simulink model "ArduinoUnoTemplate"  (R2021b)
settings: Solver=ode3  StartTime=0.0  StopTime=10  RelTol=1e-3  EnableMultiTasking=on
libraries: simulink x1, arduinolib x1
settings Model: FPTRunName=Active  ExtModeTrigDuration=2  Creator=cirie  LastModifiedBy=cirie
settings SolverCC: AlgebraicLoopSolver=TrustRegion
settings DataIOCC: LimitDataPoints=on  SaveFormat=Array
settings OptimizationCC: ExpressionDepthLimit=2147483647  LifeSpan=Inf  MaxStackSize=64
settings DebuggingCC: UnderspecifiedInitializationDetection=Classic  MergeDetectMultiDrivingBlocksExec=none  FcnCallInpInsideContextMsg=warning  AllowSymbolicDim=off  StateNameClashWarn=warning  SFUnexpectedBacktrackingDiag=warning  SFNoUnconditionalDefaultTransitionDiag=warning  SFExecutionAtInitializationDiag=none  SFMachineParentedDataDiag=warning  ArithmeticOperatorsInVariantConditions=warning
settings HardwareCC: ProdBitPerInt=16  ProdBitPerPointer=16  ProdBitPerSizeT=16  ProdBitPerPtrDiffT=16  ProdLargestAtomicFloat=None  ProdWordSize=8  ProdHWDeviceType=Atmel->AVR
settings ModelReferenceCC: PropagateSignalLabelsOutOfModel=off
settings SFSimCC: SimUseLocalCustomCode=off  CustomCodeUndefinedFunction=UseInterfaceOnly
settings RTWCC: Description=Embedded Coder  SystemTargetFile=ert.tlc  HardwareBoard=Arduino Uno  TemplateMakefile=ert_default_tmf  GenerateReport=on  RTWVerbose=off  RTWUseLocalCustomCode=off  Toolchain=Arduino AVR  BuildConfiguration=Faster Runs  LaunchReport=on
settings CodeAppCC: ForceParamTrailComments=on  OperatorAnnotations=on  StateflowObjectComments=on  MATLABSourceComments=on
settings ERTTargetCC: MultiwordLength=2048  ERTCustomFileBanners=off  SupportContinuousTime=on  SupportNonInlinedSFcns=on  RemoveResetFunc=off  SupportVariableSizeSignals=on  ModelStepFunctionPrototypeControlCompliant=off  ExtModeTransport=3  ExtModeStaticAlloc=on  ExtModeStaticAllocSize=250  ExtModeMexFile=ext_xcp  ExtModeIntrfLevel=Level2 - Open
settings ConfigComp: CovMetricSettings=dw  CovSaveCumulativeToWorkspaceVar=on  CovSaveSingleToWorkspaceVar=on  CovExternalEMLEnable=off  CovSFcnEnable=off

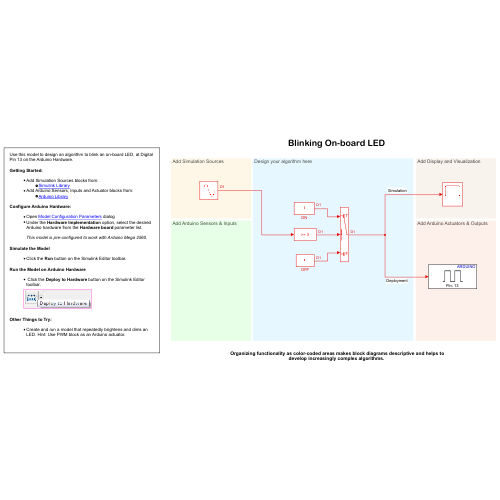
[thumbnail: Simulink's stored preview of the top-level diagram]
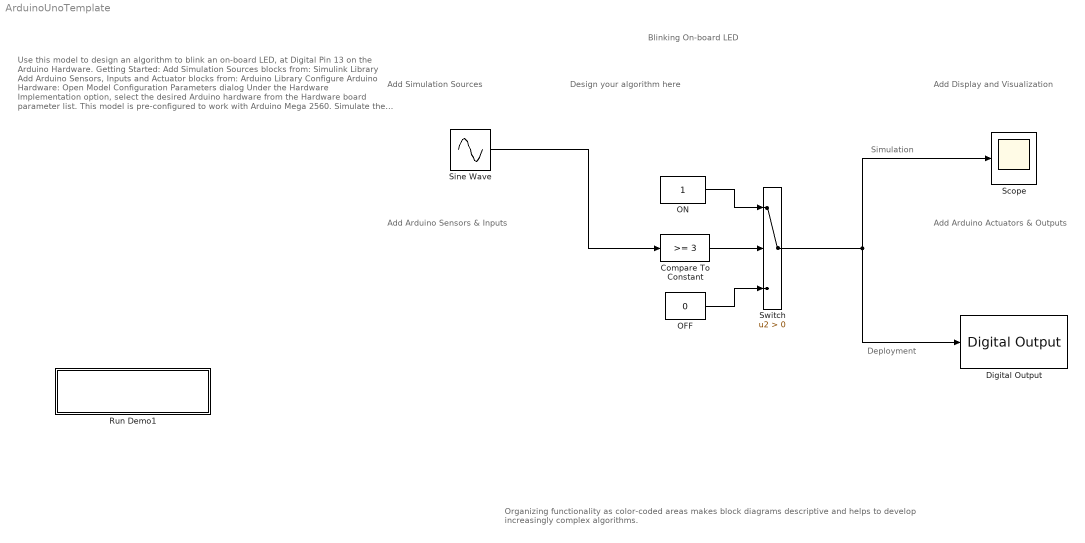
== system ArduinoUnoTemplate ==
  note: Deployment
  note: Simulation
  note: Organizing functionality as color-coded areas makes block diagrams descriptive and helps to develop increasingly complex algorithms.
  note: Add Arduino Actuators & Outputs
  note: Use this model to design an algorithm to blink an on-board LED, at Digital Pin 13 on the Arduino Hardware.
      |
      | Getting Started:
      |
      | Add Simulation Sources blocks from:
      | Simulink Library
      | Add Arduino Sensors, Inputs and Actuator blocks from:
      | Arduino Library
      |
      | Configure Arduino Hardware:
      |
      | Open Model Configuration Parameters dialog
      | Under the Hardware Implementation option, select the desired Arduino hardware from the Hardware board parameter list.
      |
      | This model is pre-configured to work with Arduino Mega 2560.
      |
      | Simulate the Model
      |
      | Click the Run button on the Simulink Editor toolbar.
      |
      | Run the Model on Arduino Hardware
      |
      | Click the Deploy to Hardware button on the Simulink Editor toolbar.
      |
      | Other Things to Try:
      |
      | Create and run a model that repeatedly brightens and dims an LED. Hint: Use PWM block as an Arduino actuator.
  note: Add Arduino Sensors & Inputs
  note: Design your algorithm here
  note: Add Display and Visualization
  note: Add Simulation Sources
  note: Blinking On-board LED
  Compare To Constant : simulink/Logic and Bit Operations/Compare To Constant  relop=>=  const=3  OutDataTypeStr=boolean
  Digital Output : arduinolib/Digital Output  pinNumber=13  Direction=output  blockPlatform=arduino
  OFF : Constant  Value=0  SampleTime=-1
  ON : Constant  SampleTime=-1
  Run Demo1 : Subsystem  Description=Controls host-side RTDX processing.
      mask Display: pic=imread('arduinoDeploytoHardware.png');image(pic);
  Scope : Scope
  Sine Wave : Sin  SineType=Sample based  Amplitude=5  SampleTime=0.1
  Switch : Switch  Criteria=u2 > Threshold
  wires:
  ON/1 -> Switch/1
  Compare To Constant/1 -> Switch/2
  OFF/1 -> Switch/3
  Sine Wave/1 -> Compare To Constant/1
  Switch/1 -> Scope/1, Digital Output/1

== system ArduinoUnoTemplate/Run Demo1 ==
